simulink library "lib_SystemDiag"  (R2017a)
settings: Solver=VariableStepAuto  StartTime=0.0  StopTime=10.0  RelTol=1e-3
settings Model: Creator=Di Russo  LastModifiedBy=Di Russo

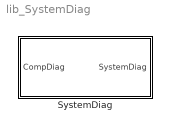
== system lib_SystemDiag ==
  SystemDiag : Subsystem

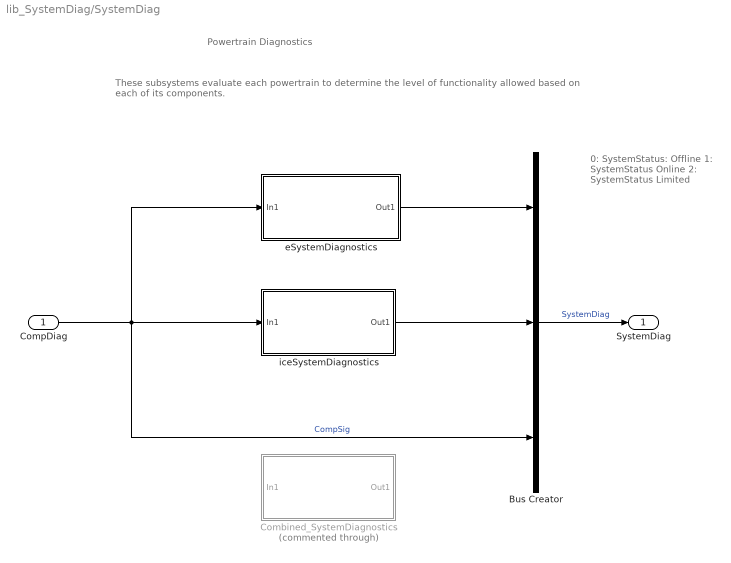
== system lib_SystemDiag/SystemDiag ==
  note: 0: SystemStatus: Offline
      | 1: SystemStatus Online
      | 2: SystemStatus Limited
  note: Powertrain Diagnostics
  note: These subsystems evaluate each powertrain to determine
      | the level of functionality allowed based on each of its components.
  CompDiag : Inport
  Bus Creator : BusCreator  Inputs=3
  Combined_SystemDiagnostics : Subsystem  Commented=through
  eSystemDiagnostics : Subsystem
  iceSystemDiagnostics : Subsystem
  SystemDiag : Outport
  wires:
  eSystemDiagnostics/1(Out1) -> Bus Creator/1
  Bus Creator/1 -> SystemDiag/1  "SystemDiag"
  CompDiag/1 -> iceSystemDiagnostics/1(In1), Bus Creator/3, eSystemDiagnostics/1(In1)  "CompSig"
  iceSystemDiagnostics/1(Out1) -> Bus Creator/2

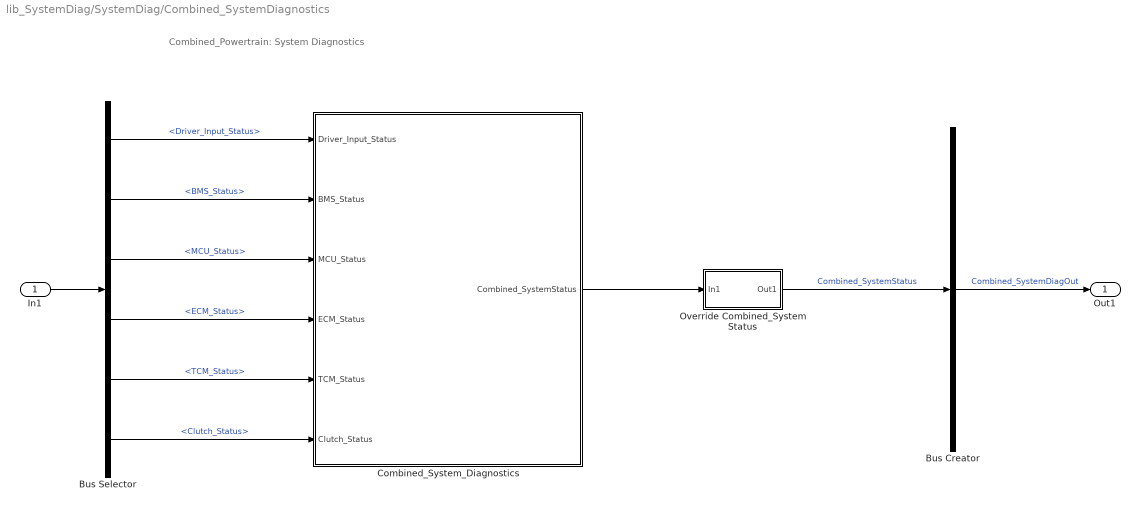
== system lib_SystemDiag/SystemDiag/Combined_SystemDiagnostics ==
  note: Combined_Powertrain: System Diagnostics
  In1 : Inport
  Bus Creator : BusCreator  Inputs=1
  Bus Selector : BusSelector  OutputSignals=Driver_Input_Status.Driver_Input_Status,BMS_Status.BMS_Status,MCU_Status.MCU_Status,ECM_Status.ECM_Status,TCM_CompDiag.TCM_Status,Clutch_Status.Clutch_Status
  Combined_System_Diagnostics : Stateflow chart  TreatAsAtomicUnit=on
  Override Combined_System Status : Subsystem
  Out1 : Outport
  wires:
  In1/1 -> Bus Selector/1
  Bus Creator/1 -> Out1/1  "Combined_SystemDiagOut"
  Override Combined_System Status/1(Out1) -> Bus Creator/1  "Combined_SystemStatus"
  Bus Selector/1 -> Combined_System_Diagnostics/1(Driver_Input_Status)  "<Driver_Input_Status>"
  Bus Selector/2 -> Combined_System_Diagnostics/2(BMS_Status)  "<BMS_Status>"
  Bus Selector/3 -> Combined_System_Diagnostics/3(MCU_Status)  "<MCU_Status>"
  Bus Selector/4 -> Combined_System_Diagnostics/4(ECM_Status)  "<ECM_Status>"
  Bus Selector/5 -> Combined_System_Diagnostics/5(TCM_Status)  "<TCM_Status>"
  Bus Selector/6 -> Combined_System_Diagnostics/6(Clutch_Status)  "<Clutch_Status>"
  Combined_System_Diagnostics/1(Combined_SystemStatus) -> Override Combined_System Status/1(In1)

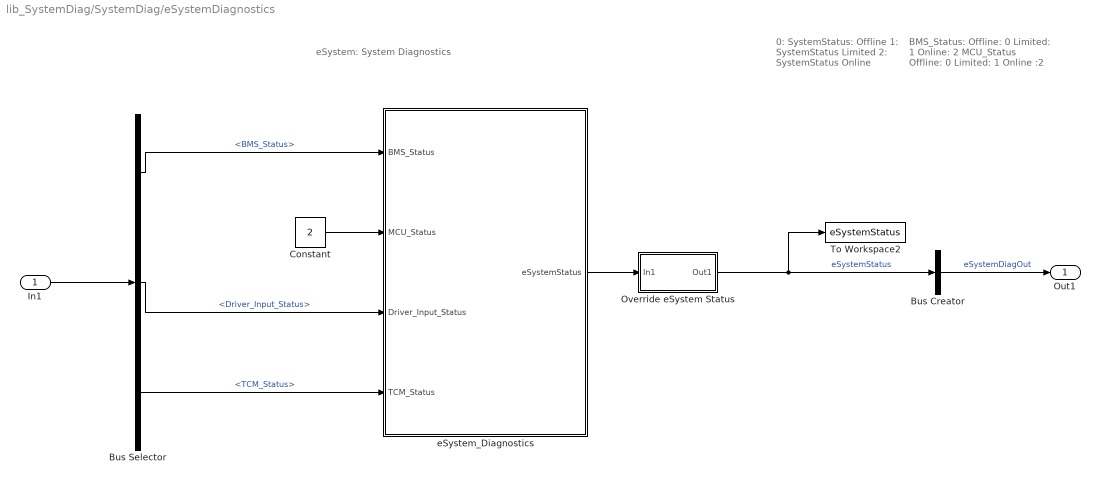
== system lib_SystemDiag/SystemDiag/eSystemDiagnostics ==
  note: BMS_Status:
      | Offline: 0
      | Limited: 1
      | Online: 2
      |
      | MCU_Status
      | Offline: 0
      | Limited: 1
      | Online :2
  note: 0: SystemStatus: Offline
      | 1: SystemStatus Limited
      | 2: SystemStatus Online
  note: eSystem: System Diagnostics
  In1 : Inport
  Bus Creator : BusCreator  Inputs=1
  Bus Selector : BusSelector  OutputSignals=BMS_Status,Driver_Input_Status,TCM_Status
  Constant : Constant  Value=2
  Override eSystem Status : Subsystem
  To Workspace2 : ToWorkspace  VariableName=eSystemStatus  SaveFormat=Timeseries  SampleTime=-1
  eSystem_Diagnostics : Stateflow chart  TreatAsAtomicUnit=on
  Out1 : Outport
  wires:
  Constant/1 -> eSystem_Diagnostics/2(MCU_Status)
  In1/1 -> Bus Selector/1
  Bus Selector/1 -> eSystem_Diagnostics/1(BMS_Status)  "<BMS_Status>"
  Bus Creator/1 -> Out1/1  "eSystemDiagOut"
  Bus Selector/2 -> eSystem_Diagnostics/3(Driver_Input_Status)  "<Driver_Input_Status>"
  Override eSystem Status/1(Out1) -> To Workspace2/1, Bus Creator/1  "eSystemStatus"
  eSystem_Diagnostics/1(eSystemStatus) -> Override eSystem Status/1(In1)
  Bus Selector/3 -> eSystem_Diagnostics/4(TCM_Status)  "<TCM_Status>"

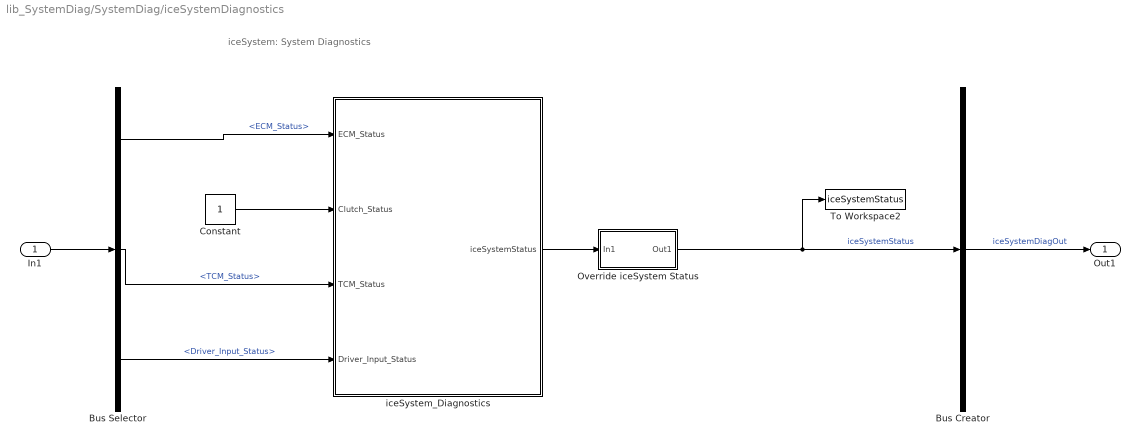
== system lib_SystemDiag/SystemDiag/iceSystemDiagnostics ==
  note: iceSystem: System Diagnostics
  In1 : Inport
  Bus Creator : BusCreator  Inputs=1
  Bus Selector : BusSelector  OutputSignals=ECM_Status,TCM_Status,Driver_Input_Status
  Constant : Constant
  Override iceSystem Status : Subsystem
  To Workspace2 : ToWorkspace  VariableName=iceSystemStatus  SaveFormat=Timeseries  SampleTime=-1
  iceSystem_Diagnostics : Stateflow chart  TreatAsAtomicUnit=on
  Out1 : Outport
  wires:
  Override iceSystem Status/1(Out1) -> To Workspace2/1, Bus Creator/1  "iceSystemStatus"
  Bus Selector/1 -> iceSystem_Diagnostics/1(ECM_Status)  "<ECM_Status>"
  Bus Creator/1 -> Out1/1  "iceSystemDiagOut"
  In1/1 -> Bus Selector/1
  Bus Selector/2 -> iceSystem_Diagnostics/3(TCM_Status)  "<TCM_Status>"
  Bus Selector/3 -> iceSystem_Diagnostics/4(Driver_Input_Status)  "<Driver_Input_Status>"
  iceSystem_Diagnostics/1(iceSystemStatus) -> Override iceSystem Status/1(In1)
  Constant/1 -> iceSystem_Diagnostics/2(Clutch_Status)

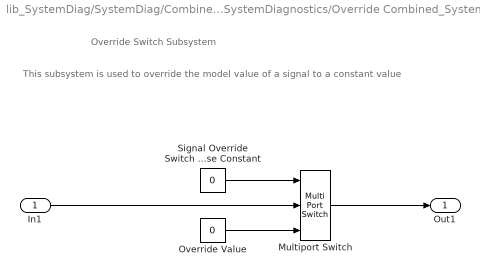
== system lib_SystemDiag/SystemDiag/Combined_SystemDiagnostics/Override Combined_System Status ==
  note: Override Switch Subsystem
  note: This subsystem is used to override the model value of a signal to a constant value
  In1 : Inport
  Multiport Switch : MultiPortSwitch  DataPortOrder=Zero-based contiguous  Inputs=2  zeroidx=on
  Override Value : Constant  Value=0  OutDataTypeStr=double
  Signal Override Switch 0 = Use Model 1 = Use Constant : Constant  Value=0
  Out1 : Outport
  wires:
  Override Value/1 -> Multiport Switch/3
  Multiport Switch/1 -> Out1/1
  In1/1 -> Multiport Switch/2
  Signal Override Switch 0 = Use Model 1 = Use Constant/1 -> Multiport Switch/1

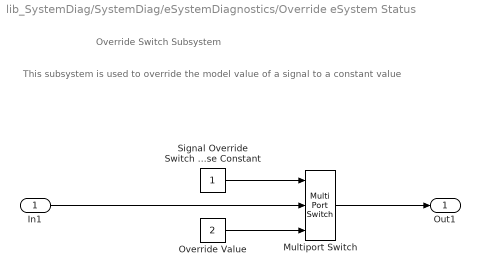
== system lib_SystemDiag/SystemDiag/eSystemDiagnostics/Override eSystem Status ==
  note: This subsystem is used to override the model value of a signal to a constant value
  note: Override Switch Subsystem
  In1 : Inport
  Multiport Switch : MultiPortSwitch  DataPortOrder=Zero-based contiguous  Inputs=2  zeroidx=on
  Override Value : Constant  Value=2  OutDataTypeStr=double
  Signal Override Switch 0 = Use Model 1 = Use Constant : Constant
  Out1 : Outport
  wires:
  Signal Override Switch 0 = Use Model 1 = Use Constant/1 -> Multiport Switch/1
  In1/1 -> Multiport Switch/2
  Multiport Switch/1 -> Out1/1
  Override Value/1 -> Multiport Switch/3

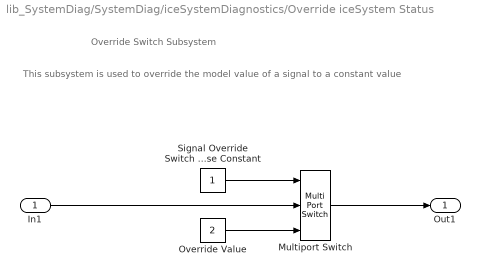
== system lib_SystemDiag/SystemDiag/iceSystemDiagnostics/Override iceSystem Status ==
  note: This subsystem is used to override the model value of a signal to a constant value
  note: Override Switch Subsystem
  In1 : Inport
  Multiport Switch : MultiPortSwitch  DataPortOrder=Zero-based contiguous  Inputs=2  zeroidx=on
  Override Value : Constant  Value=2  OutDataTypeStr=double
  Signal Override Switch 0 = Use Model 1 = Use Constant : Constant
  Out1 : Outport
  wires:
  Signal Override Switch 0 = Use Model 1 = Use Constant/1 -> Multiport Switch/1
  In1/1 -> Multiport Switch/2
  Multiport Switch/1 -> Out1/1
  Override Value/1 -> Multiport Switch/3

== stateflow chart lib_SystemDiag/SystemDiag/Combined_SystemDiagnostics/Combined_System_Diagnostics ==
  state CombinedSystem_Online
    en: Combined_SystemStatus=2
  state Combined_System_Offline
    en:Combined_SystemStatus=0
  state Combined_System_Limited
    en: Combined_SystemStatus=1
  (default) -> Combined_System_Offline
  Combined_System_Offline -> CombinedSystem_Online [order 1] : [ECM_Status==2&&Clutch_Status==1&&Driver_Input_Status==1&&TCM_Status==2&&BMS_Status==2&&MCU_Status==2]
  CombinedSystem_Online -> Combined_System_Offline [order 1] : [Clutch_Status==0||ECM_Status==0||Driver_Input_Status==0||TCM_Status==0||BMS_Status==0||MCU_Status==0]
  CombinedSystem_Online -> Combined_System_Limited [order 2] : [Driver_Input_Status==1&&Clutch_Status==1&&[ECM_Status==1||TCM_Status==1||BMS_Status==1||MCU_Status==1]]
  Combined_System_Limited -> CombinedSystem_Online [order 2] : [ECM_Status==2&&Clutch_Status==1&&Driver_Input_Status==1&&TCM_Status==2&&BMS_Status==2&&MCU_Status==2]
  Combined_System_Limited -> Combined_System_Offline [order 1] : [Clutch_Status==0||ECM_Status==0||Driver_Input_Status==0||TCM_Status==0||BMS_Status==0||MCU_Status==0]
  Combined_System_Offline -> Combined_System_Limited [order 2] : [Driver_Input_Status==1&&Clutch_Status==1&&[ECM_Status==1||TCM_Status==1||BMS_Status==1||MCU_Status==1]]
  data: Driver_Input_Status input; BMS_Status input; MCU_Status input; ECM_Status input; TCM_Status input; Clutch_Status input; Combined_SystemStatus output

== stateflow chart lib_SystemDiag/SystemDiag/eSystemDiagnostics/eSystem_Diagnostics ==
  state eSystem_Offline
    en:eSystemStatus=0;
  state eSystem_Online
    en: eSystemStatus=2;
  state eSystem_Limited
    en: eSystemStatus=1;
  (default) -> eSystem_Offline
  eSystem_Offline -> eSystem_Online [order 1] : [BMS_Status==2&&MCU_Status==2&&Driver_Input_Status==1&&TCM_Status==2]
  eSystem_Online -> eSystem_Offline [order 1] : [BMS_Status==0||MCU_Status==0||Driver_Input_Status==0||TCM_Status==0]
  eSystem_Online -> eSystem_Limited [order 2] : [Driver_Input_Status==1&&...
      | [BMS_Status==1||MCU_Status==1||...
      | TCM_Status==1]]
  eSystem_Limited -> eSystem_Online [order 2] : [BMS_Status==2&&...
      | MCU_Status==2&&...
      | Driver_Input_Status==1&&TCM_Status==2]
  eSystem_Limited -> eSystem_Offline [order 1] : [BMS_Status==0||...
      | MCU_Status==0||...
      | Driver_Input_Status==0||...
      | TCM_Status==0]
  eSystem_Offline -> eSystem_Limited [order 2] : [Driver_Input_Status==1&&...
      | [BMS_Status==1||MCU_Status==1||...
      | TCM_Status==1]]
  data: BMS_Status input; MCU_Status input; Driver_Input_Status input; TCM_Status input; eSystemStatus output

== stateflow chart lib_SystemDiag/SystemDiag/iceSystemDiagnostics/iceSystem_Diagnostics ==
  state iceSystem_Online
    en: iceSystemStatus=2;
  state iceSystem_Offline
    en:iceSystemStatus=0;
  state iceSystem_Limited
    en: iceSystemStatus=1;
  (default) -> iceSystem_Offline
  iceSystem_Offline -> iceSystem_Online [order 1] : [ECM_Status==2&&Clutch_Status==1&&Driver_Input_Status==1&&TCM_Status==2]
  iceSystem_Online -> iceSystem_Offline [order 1] : [ECM_Status==0||Clutch_Status==0||Driver_Input_Status==0||TCM_Status==0]
  iceSystem_Online -> iceSystem_Limited [order 2] : [Driver_Input_Status==1&&...
      | Clutch_Status==1&&...
      | [ECM_Status==1||TCM_Status==1]]
  iceSystem_Limited -> iceSystem_Online [order 2] : [ECM_Status==2&&...
      | Clutch_Status==1&&...
      | Driver_Input_Status==1&&TCM_Status==2]
  iceSystem_Limited -> iceSystem_Offline [order 1] : [ECM_Status==0||...
      | Clutch_Status==0||...
      | Driver_Input_Status==0||...
      | TCM_Status==0]
  iceSystem_Offline -> iceSystem_Limited [order 2] : [Driver_Input_Status==1&&...
      | Clutch_Status==1&&...
      | (ECM_Status==1||TCM_Status==1)]
  data: ECM_Status input; Clutch_Status input; TCM_Status input; Driver_Input_Status input; iceSystemStatus output
